simulink model "bicycle_model"  (R2022b)
settings: Solver=VariableStepAuto  StartTime=0.0  StopTime=20  RelTol=1e-3
model workspace (MAT data in the model file):
  L = 2
undefined symbols (not defined in the file): sigbuilder_block
settings Model: Creator=cesguti  LastModifiedBy=cesguti

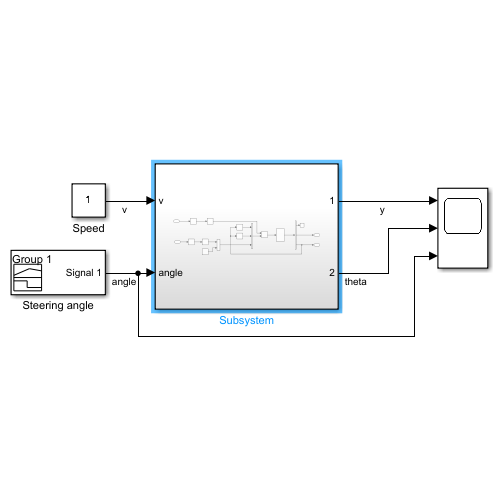
[thumbnail: Simulink's stored preview of the top-level diagram]
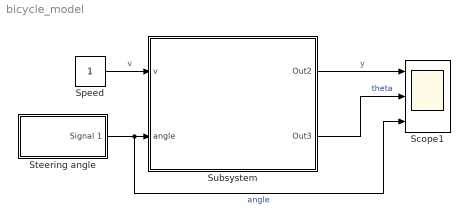
== system bicycle_model ==
  Scope1 : Scope  NumInputPorts=3
  Speed : Constant
  Steering angle : Subsystem  Tag=STV Subsys  LoadFcn=sigbuilder_block('load');  StartFcn=sigbuilder_block('start');  StopFcn=sigbuilder_block('stop');  ClipboardFcn=sigbuilder_block('clipboard');  mask(Sigbuilder block){tuvar=[0:10]}
      mask help: Simulink:masks:SigbuilderBlock_MD
      mask init:
      | if ~strcmp(get_param(bdroot(gcbh),'SimulationStatus'),'stopped') tuvar = sigbuilder_block('maskInit'); end
      settings: CopyFcn=sigbuilder_block('copy');  DeleteFcn=sigbuilder_block('delete');  ModelCloseFcn=sigbuilder_block('modelClose');  PreSaveFcn=sigbuilder_block('preSave');  PauseFcn=sigbuilder_block('pause');  ContinueFcn=sigbuilder_block('continue');  NameChangeFcn=sigbuilder_block('namechange');  OpenFcn=sigbuilder_block('open',[437.6 199.2 550.4 400 ]);  CloseFcn=sigbuilder_block('close');
      mask Display: plot(0, 0, 100, 100,[2, 2, 32, 32, 2], [68, 8, 8, 68, 68],[32, 2], [38, 38], [32, 19, 2],[53, 60, 44], [32, 17, 17, 2],[16, 16, 31, 31]);txt = getActiveGroup(gcbh);text(2, 100, txt,'verticalAlignment', 'top');
  Subsystem : Subsystem
  wires:
  Subsystem/1(Out2) -> Scope1/1  "y"
  Speed/1 -> Subsystem/1(v)  "v"
  Steering angle/1(Signal 1) -> Scope1/3, Subsystem/2(angle)  "angle"
  Subsystem/2(Out3) -> Scope1/2  "theta"

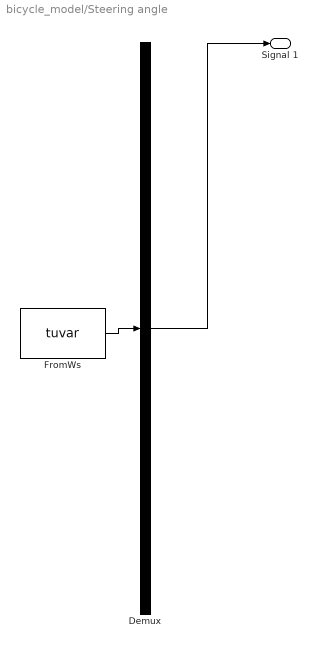
== system bicycle_model/Steering angle ==
  Demux : Demux  Tag=STV Demux  Outputs=1
      settings: DisplayOption=none
  FromWs : FromWorkspace  Tag=STV FromWs  VariableName=tuvar
      SigBuilderData=|
      | common.afterFinalStr = 'Extrapolate'
      | common.sampleTime = 0
      | dataSet.timeRange = [0 20]
      | dataSet.name = 'Group 1'
      | sbobj.Groups.Name = 'Group 1'
      | sbobj.Groups.Signals.Name = 'Signal 1'
      | sbobj.Groups.Signals.XData = [0 2.05 2.05 6.05 6.05 10 10 14.05 14.05 20]
      | sbobj.Groups.Signals.YData = [0 0 1 1 0 0 -1 -1 0 0]
      | sbobj.Groups.TimeRange = [0 20]
  Signal 1 : Outport  Tag=STV Outport
  wires:
  Demux/1 -> Signal 1/1
  FromWs/1 -> Demux/1

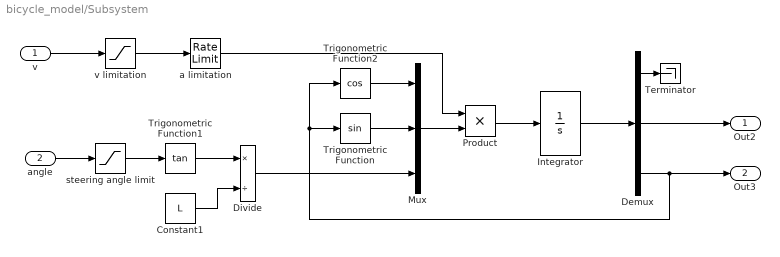
== system bicycle_model/Subsystem ==
  v : Inport
  angle : Inport  Port=2
  Constant1 : Constant  Value=L
  Demux : Demux  Outputs=3
  Divide : Product  Inputs=*/
  Integrator : Integrator
  Mux : Mux  Inputs=3
  Product : Product
  Terminator : Terminator
  Trigonometric Function : Trigonometry
  Trigonometric Function1 : Trigonometry  Operator=tan
  Trigonometric Function2 : Trigonometry  Operator=cos
  a limitation : RateLimiter  RisingSlewLimit=3  FallingSlewLimit=-3  SampleTimeMode=inherited
  steering angle limit : Saturate  UpperLimit=deg2rad(30)  LowerLimit=deg2rad(-30)
  v limitation : Saturate  UpperLimit=100  LowerLimit=-100
  Out2 : Outport
  Out3 : Outport  Port=2
  wires:
  steering angle limit/1 -> Trigonometric Function1/1
  Product/1 -> Integrator/1
  Divide/1 -> Mux/3
  Trigonometric Function/1 -> Mux/2
  v/1 -> v limitation/1
  Constant1/1 -> Divide/2
  Mux/1 -> Product/2
  Trigonometric Function1/1 -> Divide/1
  Trigonometric Function2/1 -> Mux/1
  v limitation/1 -> a limitation/1
  Demux/2 -> Out2/1
  Integrator/1 -> Demux/1
  angle/1 -> steering angle limit/1
  Demux/1 -> Terminator/1
  Demux/3 -> Trigonometric Function/1, Trigonometric Function2/1, Out3/1
  a limitation/1 -> Product/1
